simulink model "io_and_serial_telem"  (R2021a)
settings: Solver=FixedStepAuto  StartTime=0.0  StopTime=10.0  RelTol=1e-3  EnableMultiTasking=on
undefined symbols (not defined in the file or in its folder): AUX, dev, pwm_output1
libraries: px4lib x7, px4Sensorslib x3, sharedtransform x2, px4uORBlib x1, simulink x1
settings Model: ExtModeTrigDuration=10  Creator=Kawaguchi  LastModifiedBy=beket
settings SolverCC: PositivePriorityOrder=on
settings OptimizationCC: EnhancedBackFolding=on  PassReuseOutputArgsAs=Individual arguments  ZeroExternalMemoryAtStartup=off  ZeroInternalMemoryAtStartup=off  MaxStackSize=64  OptimizeBlockOrder=speed  DifferentSizesBufferReuse=on  OptimizationCustomize=off  EfficientTunableParamExpr=on
settings DebuggingCC: ParameterTunabilityLossMsg=error
settings HardwareCC: ProdBitPerPointer=32  ProdBitPerSizeT=32  ProdBitPerPtrDiffT=32  ProdLargestAtomicInteger=Long  ProdLargestAtomicFloat=Double  ProdWordSize=32  ProdLongLongMode=on  ProdHWDeviceType=ARM Compatible->ARM Cortex
settings SFSimCC: MATLABDynamicMemAlloc=off  SimTargetLang=C++
settings RTWCC: SystemTargetFile=ert.tlc  HardwareBoard=PX4 Pixhawk 4  TLCOptions="-aInlineSetEventsForThisBaseRateFcn=TLC_FALSE -aSuppressMultiTaskScheduler=TLC_FALSE  -aRateBasedStepFcn=0"  TemplateMakefile=ert_default_tmf  Toolchain=GNU Tools for PX4 Autopilots  TargetLang=C++
settings CodeAppCC: ForceParamTrailComments=on  IgnoreCustomStorageClasses=off  OperatorAnnotations=on  SimulinkDataObjDesc=on  SFDataObjDesc=on  InsertBlockDesc=on
settings ERTTargetCC: ExtModeTransport=3  ExtModeStaticAlloc=on  ExtModeStaticAllocSize=1024  ExtModeMexFile=ext_xcp  ExtModeIntrfLevel=Level2 - Open

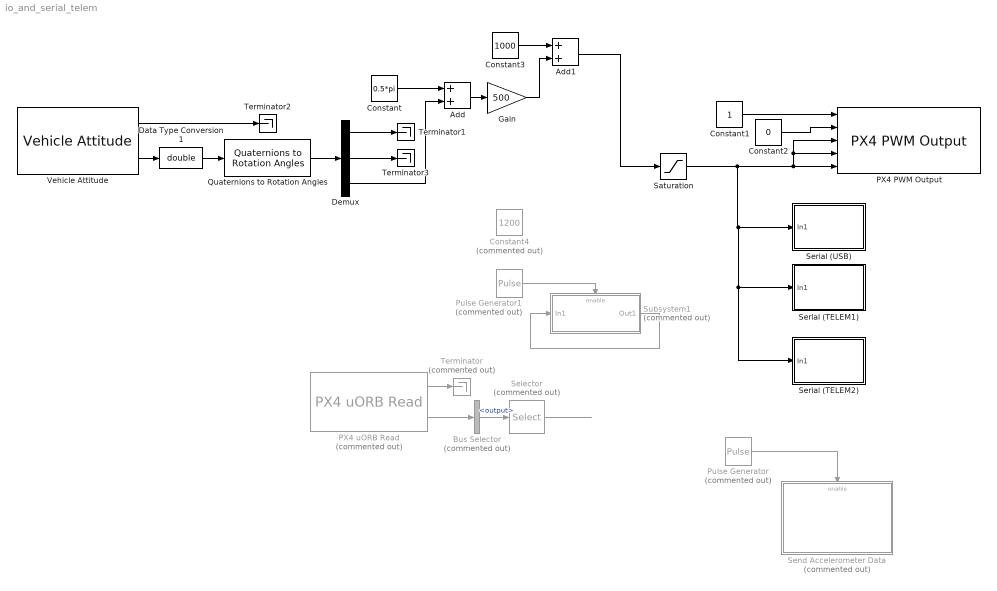
== system io_and_serial_telem ==
  Add : Sum
  Add1 : Sum
  Bus Selector : BusSelector  Commented=on  OutputSignals=output
  Constant : Constant  Value=0.5*pi
  Constant1 : Constant  OutDataTypeStr=boolean
  Constant2 : Constant  Value=0  OutDataTypeStr=boolean
  Constant3 : Constant  Value=1000
  Constant4 : Constant  Commented=on  Value=1200  OutDataTypeStr=uint16
  Data Type Conversion1 : DataTypeConversion  OutDataTypeStr=double
  Demux : Demux  Outputs=3
  Gain : Gain  Gain=500
  PX4 PWM Output : px4lib/PX4 PWM Output  pwmDevice=AUX (/dev/pwm_output1)  pwmChannel1_=on  pwmChannel2_=on  pwmChannel3_=off  pwmChannel4_=off  pwmChannel5_=on  pwmChannel6_=off  pwmChannel7_=off  pwmChannel8_=off  forceTerminateFailsafe=off  outputErrorStatus=off
      settings: SourceProductBaseCode=PX4AUTOPILOTS
  PX4 uORB Read : px4uORBlib/PX4 uORB Read  Commented=on  uORBTopic=actuator_outputs  selectInstance=actuator_outputs  SampleTime=-1  BlockingMode=off  BlockTimeout=1e-3
      settings: SourceProductBaseCode=PX4AUTOPILOTS
  Pulse Generator : DiscretePulseGenerator  Commented=on  PulseType=Time based  Period=0.1  PulseWidth=50
  Pulse Generator1 : DiscretePulseGenerator  Commented=on  PulseType=Time based  Period=1/1000  PulseWidth=50
  Quaternions to Rotation Angles : sharedtransform/Quaternions to Rotation Angles  rotationOrder=ZYX  aMode=aMode
      settings: SourceProductBaseCode=AE,PW,DR,MT,UV,VE
  Saturation : Saturate  UpperLimit=2000  LowerLimit=1000  OutDataTypeStr=uint16
  Selector : Selector  Commented=on  InputPortWidth=16  IndexOptions=Index vector (dialog)  Indices=[1 2]  OutputSizes=1
  Send Accelerometer Data : Subsystem  Commented=on
  Serial (TELEM1) : Subsystem
  Serial (TELEM2) : Subsystem
  Serial (USB) : Subsystem
  Subsystem1 : Subsystem  Commented=on
  Terminator : Terminator  Commented=on
  Terminator1 : Terminator
  Terminator2 : Terminator
  Terminator3 : Terminator
  Vehicle Attitude : px4Sensorslib/Vehicle Attitude  rollRate=off  pitchRate=off  yawRate=off  quaternion=on  uorbTimeStamp=off  BlockingMode=off  BlockTimeout=0.001  sampleTime=1/250
      settings: SourceProductBaseCode=PX4AUTOPILOTS
  wires:
  Pulse Generator/1 -> Send Accelerometer Data/Enable
  Constant1/1 -> PX4 PWM Output/1
  Data Type Conversion1/1 -> Quaternions to Rotation Angles/1
  Vehicle Attitude/1 -> Terminator2/1
  Vehicle Attitude/2 -> Data Type Conversion1/1
  Quaternions to Rotation Angles/1 -> Demux/1
  Demux/3 -> Add/2
  Demux/1 -> Terminator1/1
  Demux/2 -> Terminator3/1
  Constant2/1 -> PX4 PWM Output/2
  Constant/1 -> Add/1
  Add/1 -> Gain/1
  Constant3/1 -> Add1/1
  Gain/1 -> Add1/2
  PX4 uORB Read/1 -> Terminator/1
  PX4 uORB Read/2 -> Bus Selector/1
  Selector/1 -> ?
  Bus Selector/1 -> Selector/1  "<output>"
  Add1/1 -> Saturation/1
  Pulse Generator1/1 -> Subsystem1/Enable
  Subsystem1/1(Out1) -> Subsystem1/1(In1)
  Saturation/1 -> PX4 PWM Output/5, PX4 PWM Output/4, PX4 PWM Output/3, Serial (TELEM2)/1(In1), Serial (TELEM1)/1(In1), Serial (USB)/1(In1)

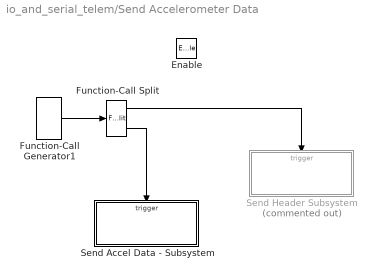
== system io_and_serial_telem/Send Accelerometer Data ==
  Enable : EnablePort
  Function-Call Generator1 : simulink/Ports & Subsystems/Function-Call Generator  sample_time=-1  numberOfIterations=1  DisallowWideOutput=off
  Function-Call Split : FunctionCallSplit  IconShape=distinctive  NumOutputPorts=2  OutputPortLayout=default
  Send Accel Data - Subsystem : Subsystem  TreatAsAtomicUnit=on
  Send Header Subsystem : Subsystem  Commented=on  TreatAsAtomicUnit=on
  wires:
  Function-Call Generator1/1 -> Function-Call Split/1
  Function-Call Split/1 -> Send Header Subsystem/Trigger
  Function-Call Split/2 -> Send Accel Data - Subsystem/Trigger

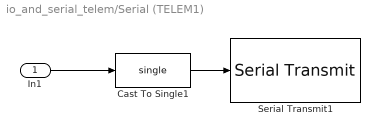
== system io_and_serial_telem/Serial (TELEM1) ==
  In1 : Inport
  Cast To Single1 : DataTypeConversion  OutDataTypeStr=single
  Serial Transmit1 : px4lib/Serial Transmit  SCIModule=/dev/ttyS1
      settings: SourceProductBaseCode=PX4AUTOPILOTS
  wires:
  Cast To Single1/1 -> Serial Transmit1/1
  In1/1 -> Cast To Single1/1

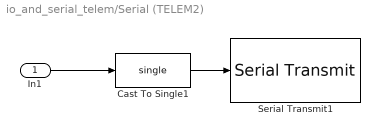
== system io_and_serial_telem/Serial (TELEM2) ==
  In1 : Inport
  Cast To Single1 : DataTypeConversion  OutDataTypeStr=single
  Serial Transmit1 : px4lib/Serial Transmit  SCIModule=/dev/ttyS2
      settings: SourceProductBaseCode=PX4AUTOPILOTS
  wires:
  Cast To Single1/1 -> Serial Transmit1/1
  In1/1 -> Cast To Single1/1

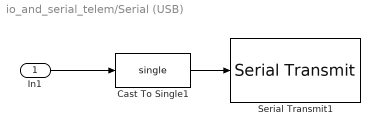
== system io_and_serial_telem/Serial (USB) ==
  In1 : Inport
  Cast To Single1 : DataTypeConversion  OutDataTypeStr=single
  Serial Transmit1 : px4lib/Serial Transmit  SCIModule=/dev/ttyACM0
      settings: SourceProductBaseCode=PX4AUTOPILOTS
  wires:
  Cast To Single1/1 -> Serial Transmit1/1
  In1/1 -> Cast To Single1/1

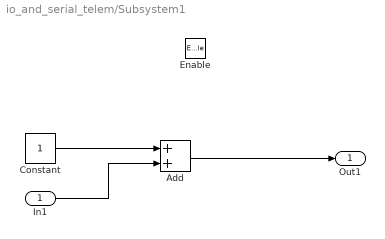
== system io_and_serial_telem/Subsystem1 ==
  In1 : Inport
  Enable : EnablePort
  Add : Sum
  Constant : Constant
  Out1 : Outport
  wires:
  Constant/1 -> Add/1
  Add/1 -> Out1/1
  In1/1 -> Add/2

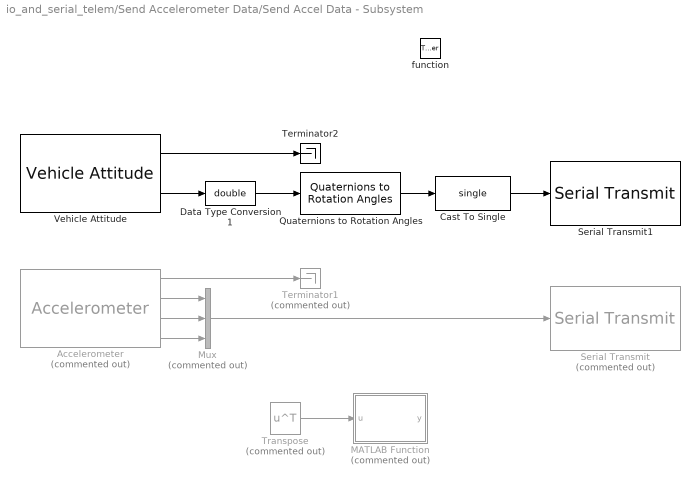
== system io_and_serial_telem/Send Accelerometer Data/Send Accel Data - Subsystem ==
  function : TriggerPort  TriggerType=function-call  VariantControl=Variant
  Accelerometer : px4Sensorslib/Accelerometer  Commented=on  uorbTimeStamp=off  BlockingMode=off  BlockTimeout=1e-3  sampleTime=-1
      settings: SourceProductBaseCode=PX4AUTOPILOTS
  Cast To Single : DataTypeConversion  OutDataTypeStr=single
  Data Type Conversion1 : DataTypeConversion  OutDataTypeStr=double
  MATLAB Function : MATLAB Function  Commented=on  TreatAsAtomicUnit=on
  Mux : Mux  Commented=on  Inputs=3
  Quaternions to Rotation Angles : sharedtransform/Quaternions to Rotation Angles  rotationOrder=ZYX  aMode=aMode
      settings: SourceProductBaseCode=AE,PW,DR,MT,UV,VE
  Serial Transmit : px4lib/Serial Transmit  Commented=on  SCIModule=/dev/ttyACM0
      settings: SourceProductBaseCode=PX4AUTOPILOTS
  Serial Transmit1 : px4lib/Serial Transmit  SCIModule=/dev/ttyACM0
      settings: SourceProductBaseCode=PX4AUTOPILOTS
  Terminator1 : Terminator  Commented=on
  Terminator2 : Terminator
  Transpose : Math  Commented=on  Operator=transpose  SaturateOnIntegerOverflow=on
  Vehicle Attitude : px4Sensorslib/Vehicle Attitude  rollRate=off  pitchRate=off  yawRate=off  quaternion=on  uorbTimeStamp=off  BlockingMode=off  BlockTimeout=0.001  sampleTime=-1
      settings: SourceProductBaseCode=PX4AUTOPILOTS
  wires:
  Accelerometer/1 -> Terminator1/1
  Accelerometer/2 -> Mux/1
  Accelerometer/3 -> Mux/2
  Accelerometer/4 -> Mux/3
  Mux/1 -> Serial Transmit/1
  Transpose/1 -> MATLAB Function/1(u)
  Data Type Conversion1/1 -> Quaternions to Rotation Angles/1
  Vehicle Attitude/2 -> Data Type Conversion1/1
  Vehicle Attitude/1 -> Terminator2/1
  Quaternions to Rotation Angles/1 -> Cast To Single/1
  Cast To Single/1 -> Serial Transmit1/1

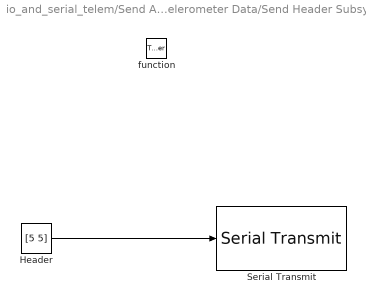
== system io_and_serial_telem/Send Accelerometer Data/Send Header Subsystem ==
  function : TriggerPort  TriggerType=function-call  VariantControl=Variant
  Header : Constant  Value=[5 5]  OutDataTypeStr=uint8  SampleTime=-1
  Serial Transmit : px4lib/Serial Transmit  SCIModule=/dev/ttyACM0
      settings: SourceProductBaseCode=PX4AUTOPILOTS
  wires:
  Header/1 -> Serial Transmit/1

== matlab function io_and_serial_telem/Send Accelerometer Data/Send Accel Data - Subsystem/MATLAB Function ==
  data: u input; y output
function y = fcn(u)
y = char(u);
